simulink model "wahadlo_z_magnesami"  (Simulink 7.3)
settings: Solver=ode45  StartTime=0.0  StopTime=inf  MaxStep=0.01  RelTol=1e-3
libraries: simulink x1
settings Model: Creator=mszubert  LastModifiedBy=psoltysiak

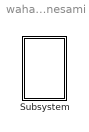
== system wahadlo_z_magnesami ==
  Subsystem : Subsystem  mask{k=0.5, m=5, g=9.81, l=100}
      mask prompts: k "hamowanie"; m "masa"; g "grawitacja"; l "dlugosc"

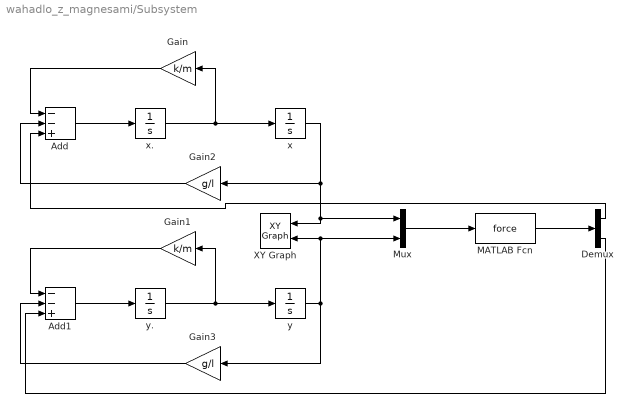
== system wahadlo_z_magnesami/Subsystem ==
  Add : Sum  Inputs=--+  OutDataType=fixdt(1, 16)  OutScaling=2^-10
  Add1 : Sum  Inputs=--+  OutDataType=fixdt(1, 16)  OutScaling=2^-10
  Demux : Demux  Outputs=2
  Gain : Gain  Gain=k/m  ParameterDataType=fixdt(1, 16)  ParameterScaling=2^0  OutDataType=fixdt(1, 16)  OutScaling=2^0
  Gain1 : Gain  Gain=k/m  ParameterDataType=fixdt(1, 16)  ParameterScaling=2^0  OutDataType=fixdt(1, 16)  OutScaling=2^0
  Gain2 : Gain  Gain=g/l  ParameterDataType=fixdt(1, 16)  ParameterScaling=2^0  OutDataType=fixdt(1, 16)  OutScaling=2^0
  Gain3 : Gain  Gain=g/l  ParameterDataType=fixdt(1, 16)  ParameterScaling=2^0  OutDataType=fixdt(1, 16)  OutScaling=2^0
  MATLAB Fcn : MATLABFcn  MATLABFcn=force
  Mux : Mux  Inputs=2
  XY Graph : simulink/Sinks/XY Graph  SystemSampleTime=-1  xmin=-1  xmax=2  ymin=-2  ymax=1  st=-1
  x : Integrator
  x. : Integrator
  y : Integrator
  y. : Integrator
  wires:
  x./1 -> x/1, Gain/1
  x/1 -> Gain2/1, Mux/1, XY Graph/1
  Gain/1 -> Add/1
  Add/1 -> x./1
  y./1 -> y/1, Gain1/1
  y/1 -> Gain3/1, Mux/2, XY Graph/2
  Gain1/1 -> Add1/1
  Add1/1 -> y./1
  Mux/1 -> MATLAB Fcn/1
  MATLAB Fcn/1 -> Demux/1
  Gain3/1 -> Add1/2
  Demux/2 -> Add1/3
  Gain2/1 -> Add/2
  Demux/1 -> Add/3
